simulink library "eomlib"  (R2023b)
settings: Solver=ode45  StartTime=0.0  StopTime=10.0  RelTol=1e-3
undefined symbols (not defined in the file or in its folder): StatesInp
libraries: Cross_Product_3D_lib x2, Euler_to_DCM_lib x1, EulerDot_lib x1, Form_Inertia_Matrix_lib x1, $bdroot x1, simulink x1
settings Model: Creator=cox  LastModifiedBy=suvo
settings SolverCC: AlgebraicLoopSolver=TrustRegion
settings DataIOCC: LimitDataPoints=on  SaveFormat=Array  SignalLoggingSaveFormat=ModelDataLogs  ReturnWorkspaceOutputs=off
settings OptimizationCC: BlockReduction=off  BooleanDataType=off  ExpressionDepthLimit=2147483647  LifeSpan=inf
settings DebuggingCC: SaveWithParameterizedLinksMsg=none  UnderspecifiedInitializationDetection=Classic  MergeDetectMultiDrivingBlocksExec=none  SignalResolutionControl=TryResolveAllWithWarning  FcnCallInpInsideContextMsg=warning  UnconnectedInputMsg=warning  UnconnectedOutputMsg=warning  UnconnectedLineMsg=warning  StateNameClashWarn=warning  SFUnexpectedBacktrackingDiag=warning  SFNoUnconditionalDefaultTransitionDiag=warning  SFExecutionAtInitializationDiag=none  ArithmeticOperatorsInVariantConditions=warning
settings HardwareCC: ProdBitPerPointer=32  ProdBitPerSizeT=32  ProdBitPerPtrDiffT=32  ProdLargestAtomicFloat=None  ProdIntDivRoundTo=Undefined  ProdEndianess=Unspecified  ProdWordSize=32  ProdHWDeviceType=32-bit Generic  TargetUnknown=on
settings ModelReferenceCC: PropagateSignalLabelsOutOfModel=off
settings SFSimCC: SimUseLocalCustomCode=off  CustomCodeUndefinedFunction=UseInterfaceOnly
settings RTWCC: RTWUseLocalCustomCode=off
settings CodeAppCC: StateflowObjectComments=on
settings GRTTargetCC: TargetLangStandard=C89/C90 (ANSI)  CombineOutputUpdateFcns=off  GRTInterface=on
settings ConfigComp: CovMetricSettings=dw  CovSaveCumulativeToWorkspaceVar=on  CovSaveSingleToWorkspaceVar=on

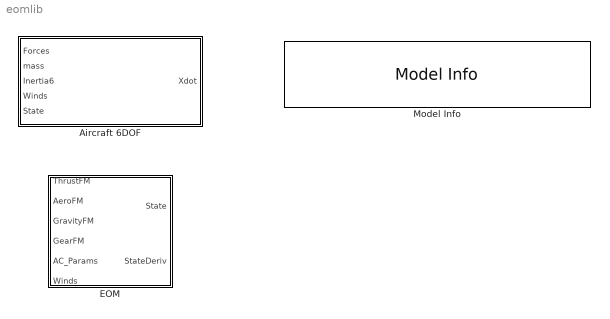
== system eomlib ==
  Aircraft 6DOF : Subsystem  mask{UnitOfLength=ft}
      mask prompts: UnitOfLength "Length Unit"
      mask help:
      | Six Degree of Freedom Aircraft Simulation
      |
      | Input forces are both linear forces and torques -> [Fx Fy Fz Tl Tm Tn].
      | Inertia6 is a vector [Ixx Iyy Izz  Ixz Iyz Ixy], all positive
      | State Vector is [Vb pqr LatLonAlt PhiThetaPsi]
      mask init:
      | if (UnitOfLength==1), % ft
      |     Re=6.37043246e+06/.3048;
      | elseif (UnitOfLength==2), % m
      |     Re=6.37043246e+06;
      | end
      mask TypeOptions UnitOfLength: ft | meters
  EOM : Subsystem
  Model Info : simulink/Model-Wide Utilities/Model Info  Frame=on  DisplayStringWithTags=|  HorizontalTextAlignment=Center  LeftAlignmentValue=0.5
      | Equations of Motion Library
      | Subversion Info: %<ModelVersion>
      | Last modified by %<LastModifiedBy> on %<LastModificationDate>

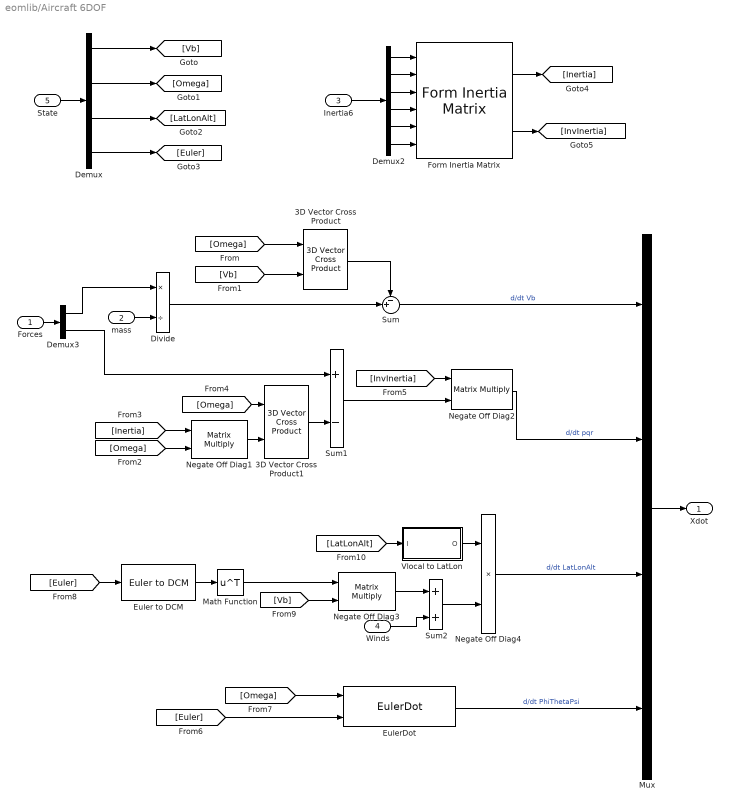
== system eomlib/Aircraft 6DOF ==
  Forces : Inport  PortDimensions=6
  mass : Inport  Port=2  PortDimensions=1
  Inertia6 : Inport  Port=3  PortDimensions=6
  Winds : Inport  Port=4
  State : Inport  Port=5  PortDimensions=12
  3D Vector Cross Product : Cross_Product_3D_lib/3D Vector Cross Product  SystemSampleTime=-1
  3D Vector Cross Product1 : Cross_Product_3D_lib/3D Vector Cross Product  SystemSampleTime=-1
  Demux : Demux  Outputs=[3 3 3 3]
  Demux2 : Demux  Outputs=6
  Demux3 : Demux  Outputs=[3 3]
  Divide : Product  Inputs=*/
  Euler to DCM : Euler_to_DCM_lib/Euler to DCM  SystemSampleTime=-1
  EulerDot : EulerDot_lib/EulerDot  SystemSampleTime=-1
  Form Inertia Matrix : Form_Inertia_Matrix_lib/Form Inertia Matrix  SystemSampleTime=-1
  Math Function : Math  Operator=transpose  SignedPower=on
  Mux : Mux
  Negate Off Diag1 : Product  Inputs=**  Multiplication=Matrix(*)
  Negate Off Diag2 : Product  Inputs=**  Multiplication=Matrix(*)
  Negate Off Diag3 : Product  Inputs=**  Multiplication=Matrix(*)
  Negate Off Diag4 : Product  Inputs=**
  Sum : Sum  Inputs=-+|  SaturateOnIntegerOverflow=on
  Sum1 : Sum  Inputs=+-  SaturateOnIntegerOverflow=on
  Sum2 : Sum
  Vlocal to LatLon : Subsystem
  Xdot : Outport
  wires:
  Mux/1 -> Xdot/1
  Math Function/1 -> Negate Off Diag3/1
  Demux/4 -> [Euler]
  Demux/3 -> [LatLonAlt]
  Demux/2 -> [Omega]
  Demux/1 -> [Vb]
  State/1 -> Demux/1
  Divide/1 -> Sum/2
  3D Vector Cross Product/1 -> Sum/1
  Negate Off Diag4/1 -> Mux/3  "d/dt LatLonAlt"
  Vlocal to LatLon/1(O) -> Negate Off Diag4/1
  [LatLonAlt] -> Vlocal to LatLon/1(I)
  [Vb] -> Negate Off Diag3/2
  Euler to DCM/1 -> Math Function/1
  [Euler] -> Euler to DCM/1
  [Omega] -> EulerDot/1
  [Euler] -> EulerDot/2
  Negate Off Diag2/1 -> Mux/2  "d/dt pqr"
  [InvInertia] -> Negate Off Diag2/1
  Sum1/1 -> Negate Off Diag2/2
  3D Vector Cross Product1/1 -> Sum1/2
  [Omega] -> 3D Vector Cross Product1/1
  Negate Off Diag1/1 -> 3D Vector Cross Product1/2
  [Inertia] -> Negate Off Diag1/1
  [Omega] -> Negate Off Diag1/2
  [Vb] -> 3D Vector Cross Product/2
  [Omega] -> 3D Vector Cross Product/1
  Demux3/2 -> Sum1/1
  mass/1 -> Divide/2
  Demux3/1 -> Divide/1
  Forces/1 -> Demux3/1
  Sum/1 -> Mux/1  "d/dt Vb"
  EulerDot/1 -> Mux/4  "d/dt PhiThetaPsi"
  Demux2/1 -> Form Inertia Matrix/1
  Demux2/2 -> Form Inertia Matrix/2
  Demux2/3 -> Form Inertia Matrix/3
  Demux2/4 -> Form Inertia Matrix/4
  Inertia6/1 -> Demux2/1
  Form Inertia Matrix/2 -> [InvInertia]
  Form Inertia Matrix/1 -> [Inertia]
  Demux2/5 -> Form Inertia Matrix/5
  Demux2/6 -> Form Inertia Matrix/6
  Negate Off Diag3/1 -> Sum2/1
  Sum2/1 -> Negate Off Diag4/2
  Winds/1 -> Sum2/2

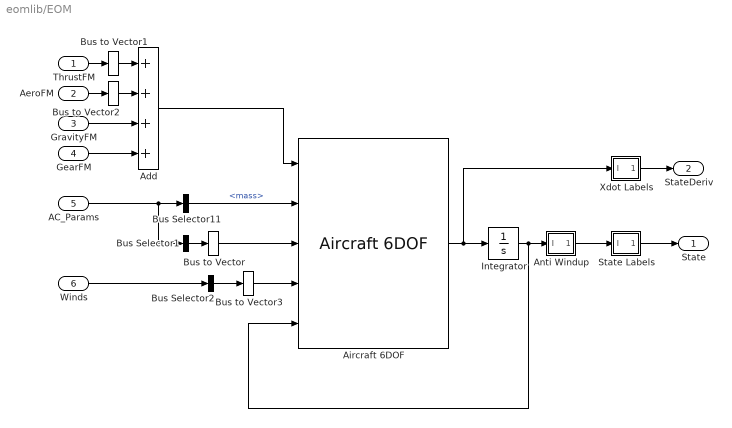
== system eomlib/EOM ==
  ThrustFM : Inport
  AeroFM : Inport  Port=2
  GravityFM : Inport  Port=3
  GearFM : Inport  Port=4
  AC_Params : Inport  Port=5
  Winds : Inport  Port=6
  Add : Sum  Inputs=++++
  Aircraft 6DOF : $bdroot/Aircraft 6DOF  SystemSampleTime=-1  UnitOfLength=ft
  Anti Windup : Subsystem
  Bus Selector1 : BusSelector  OutputSignals=Ixx,Iyy,Izz,Ixz,Iyz,Ixy  OutputAsBus=on
  Bus Selector11 : BusSelector  OutputSignals=mass
  Bus Selector2 : BusSelector  OutputSignals=NorthWind,EastWind,VerticalWind  OutputAsBus=on
  Bus to Vector{,1..3} (4 alike) : BusToVector
  Integrator : Integrator  InitialCondition=StatesInp
  State Labels : Subsystem
  Xdot Labels : Subsystem
  State : Outport
  StateDeriv : Outport  Port=2
  wires:
  AC_Params/1 -> Bus Selector11/1, Bus Selector1/1
  Bus Selector11/1 -> Aircraft 6DOF/2  "<mass>"
  Integrator/1 -> Anti Windup/1(I), Aircraft 6DOF/5
  Anti Windup/1(O) -> State Labels/1(I)
  Aircraft 6DOF/1 -> Integrator/1, Xdot Labels/1(I)
  Bus Selector1/1 -> Bus to Vector/1
  Xdot Labels/1(O) -> StateDeriv/1
  Add/1 -> Aircraft 6DOF/1
  GravityFM/1 -> Add/3
  GearFM/1 -> Add/4
  Bus to Vector/1 -> Aircraft 6DOF/3
  State Labels/1(O) -> State/1
  AeroFM/1 -> Bus to Vector2/1
  ThrustFM/1 -> Bus to Vector1/1
  Bus to Vector1/1 -> Add/1
  Bus to Vector2/1 -> Add/2
  Bus to Vector3/1 -> Aircraft 6DOF/4
  Winds/1 -> Bus Selector2/1
  Bus Selector2/1 -> Bus to Vector3/1

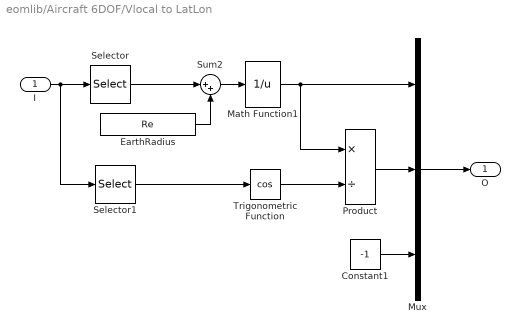
== system eomlib/Aircraft 6DOF/Vlocal to LatLon ==
  I : Inport
  Constant1 : Constant  Value=-1
  "EarthRadius " : Constant  Value=Re
  Math Function1 : Math  Operator=reciprocal  SignedPower=on
  Mux : Mux  Inputs=3
  Product : Product  Inputs=*/  RndMeth=Zero
  Selector : Selector  InputPortWidth=3  IndexOptions=Index vector (dialog)  Indices=3  OutputSizes=1
  Selector1 : Selector  InputPortWidth=3  IndexOptions=Index vector (dialog)  Indices=1  OutputSizes=1
  Sum2 : Sum  Inputs=|++
  Trigonometric Function : Trigonometry  Operator=cos
  O : Outport
  wires:
  Selector1/1 -> Trigonometric Function/1
  Mux/1 -> O/1
  I/1 -> Selector1/1, Selector/1
  Selector/1 -> Sum2/1
  Constant1/1 -> Mux/3
  Product/1 -> Mux/2
  Math Function1/1 -> Mux/1, Product/1
  Trigonometric Function/1 -> Product/2
  Sum2/1 -> Math Function1/1
  "EarthRadius "/1 -> Sum2/2

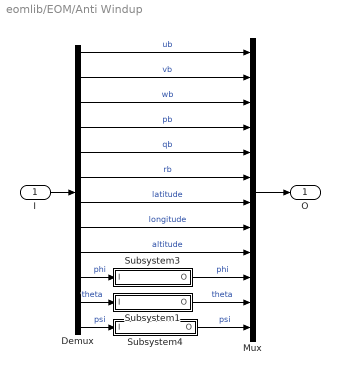
== system eomlib/EOM/Anti Windup ==
  I : Inport
  Demux : Demux  Outputs=12
      settings: DisplayOption=none
  Mux : Mux  Inputs=12
  Subsystem1 : Subsystem
      mask Display: disp('no windup 180')
  Subsystem3 : Subsystem
      mask Display: disp('no windup 180')
  Subsystem4 : Subsystem
      mask Display: disp('no windup 360')
  O : Outport
  wires:
  Demux/12 -> Subsystem4/1(I)  "psi"
  Demux/9 -> Mux/9  "altitude"
  Demux/8 -> Mux/8  "longitude"
  Demux/7 -> Mux/7  "latitude"
  Demux/6 -> Mux/6  "rb"
  Demux/5 -> Mux/5  "qb"
  Demux/4 -> Mux/4  "pb"
  Demux/3 -> Mux/3  "wb"
  Demux/2 -> Mux/2  "vb"
  Demux/1 -> Mux/1  "ub"
  I/1 -> Demux/1
  Subsystem3/1(O) -> Mux/10  "phi"
  Subsystem1/1(O) -> Mux/11  "theta"
  Subsystem4/1(O) -> Mux/12  "psi"
  Demux/10 -> Subsystem3/1(I)  "phi"
  Demux/11 -> Subsystem1/1(I)  "theta"
  Mux/1 -> O/1

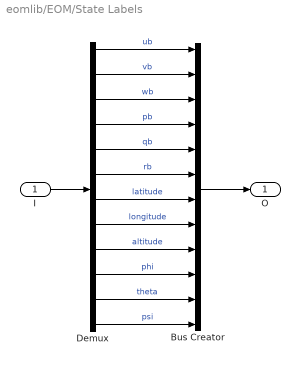
== system eomlib/EOM/State Labels ==
  I : Inport
  Bus Creator : BusCreator  Inputs=12
  Demux : Demux  Outputs=12
      settings: DisplayOption=none
  O : Outport
  wires:
  Bus Creator/1 -> O/1
  Demux/11 -> Bus Creator/11  "theta"
  Demux/10 -> Bus Creator/10  "phi"
  I/1 -> Demux/1
  Demux/1 -> Bus Creator/1  "ub"
  Demux/2 -> Bus Creator/2  "vb"
  Demux/3 -> Bus Creator/3  "wb"
  Demux/4 -> Bus Creator/4  "pb"
  Demux/5 -> Bus Creator/5  "qb"
  Demux/6 -> Bus Creator/6  "rb"
  Demux/7 -> Bus Creator/7  "latitude"
  Demux/8 -> Bus Creator/8  "longitude"
  Demux/9 -> Bus Creator/9  "altitude"
  Demux/12 -> Bus Creator/12  "psi"

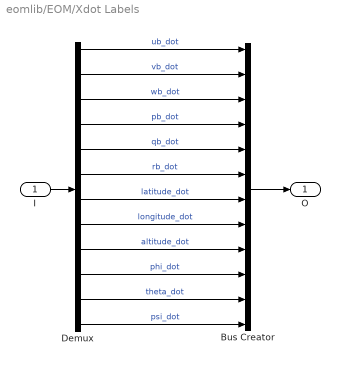
== system eomlib/EOM/Xdot Labels ==
  I : Inport
  Bus Creator : BusCreator  Inputs=12
  Demux : Demux  Outputs=12
      settings: DisplayOption=none
  O : Outport
  wires:
  Demux/12 -> Bus Creator/12  "psi_dot"
  Demux/9 -> Bus Creator/9  "altitude_dot"
  Demux/8 -> Bus Creator/8  "longitude_dot"
  Demux/7 -> Bus Creator/7  "latitude_dot"
  Demux/6 -> Bus Creator/6  "rb_dot"
  Demux/5 -> Bus Creator/5  "qb_dot"
  Demux/4 -> Bus Creator/4  "pb_dot"
  Demux/3 -> Bus Creator/3  "wb_dot"
  Demux/2 -> Bus Creator/2  "vb_dot"
  Demux/1 -> Bus Creator/1  "ub_dot"
  I/1 -> Demux/1
  Demux/10 -> Bus Creator/10  "phi_dot"
  Demux/11 -> Bus Creator/11  "theta_dot"
  Bus Creator/1 -> O/1

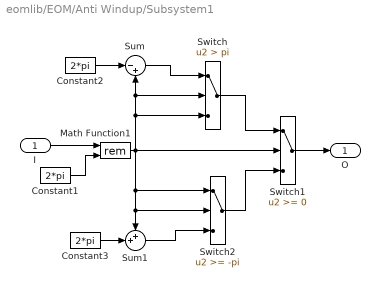
== system eomlib/EOM/Anti Windup/Subsystem1 ==
  I : Inport
  Constant1 : Constant  Value=2*pi
  Constant2 : Constant  Value=2*pi
  Constant3 : Constant  Value=2*pi
  Math Function1 : Math  Operator=rem  SignedPower=on
  Sum : Sum  Inputs=|-+  SaturateOnIntegerOverflow=on
  Sum1 : Sum  Inputs=++|  SaturateOnIntegerOverflow=on
  Switch : Switch  Criteria=u2 > Threshold  Threshold=pi  InputSameDT=off
  Switch1 : Switch  InputSameDT=off
  Switch2 : Switch  Threshold=-pi  InputSameDT=off
  O : Outport
  wires:
  Constant1/1 -> Math Function1/2
  I/1 -> Math Function1/1
  Math Function1/1 -> Switch/2, Sum/2, Switch/3, Switch2/1, Switch2/2, Sum1/1, Switch1/2
  Constant2/1 -> Sum/1
  Sum/1 -> Switch/1
  Constant3/1 -> Sum1/2
  Sum1/1 -> Switch2/3
  Switch2/1 -> Switch1/3
  Switch/1 -> Switch1/1
  Switch1/1 -> O/1

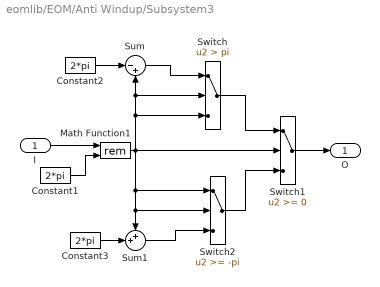
== system eomlib/EOM/Anti Windup/Subsystem3 ==
  I : Inport
  Constant1 : Constant  Value=2*pi
  Constant2 : Constant  Value=2*pi
  Constant3 : Constant  Value=2*pi
  Math Function1 : Math  Operator=rem  SignedPower=on
  Sum : Sum  Inputs=|-+  SaturateOnIntegerOverflow=on
  Sum1 : Sum  Inputs=++|  SaturateOnIntegerOverflow=on
  Switch : Switch  Criteria=u2 > Threshold  Threshold=pi  InputSameDT=off
  Switch1 : Switch  InputSameDT=off
  Switch2 : Switch  Threshold=-pi  InputSameDT=off
  O : Outport
  wires:
  Constant1/1 -> Math Function1/2
  I/1 -> Math Function1/1
  Math Function1/1 -> Switch/2, Sum/2, Switch/3, Switch2/1, Switch2/2, Sum1/1, Switch1/2
  Constant2/1 -> Sum/1
  Sum/1 -> Switch/1
  Constant3/1 -> Sum1/2
  Sum1/1 -> Switch2/3
  Switch2/1 -> Switch1/3
  Switch/1 -> Switch1/1
  Switch1/1 -> O/1

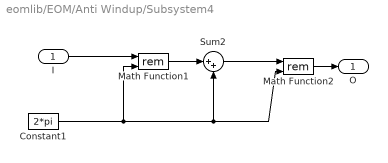
== system eomlib/EOM/Anti Windup/Subsystem4 ==
  I : Inport
  Constant1 : Constant  Value=2*pi
  Math Function1 : Math  Operator=rem  SignedPower=on
  Math Function2 : Math  Operator=rem  SignedPower=on
  Sum2 : Sum  Inputs=|++  SaturateOnIntegerOverflow=on
  O : Outport
  wires:
  Math Function2/1 -> O/1
  Math Function1/1 -> Sum2/1
  Sum2/1 -> Math Function2/1
  I/1 -> Math Function1/1
  Constant1/1 -> Sum2/2, Math Function2/2, Math Function1/2
